simulink library "THB_fixed_T"  (Simulink 8.2)
settings: Solver=ode45  StartTime=0.0  StopTime=10.0  RelTol=1e-3
libraries: carnot x1
settings Model: Creator=lena.frank  LastModifiedBy=awohlfei

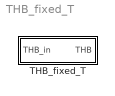
== system THB_fixed_T ==
  THB_fixed_T : Subsystem  InitFcn=load('THB.mat');  mask(set temperature in THB){t=60}
      mask prompts: t "temperature in degree Celsuis"
      mask help: Set a constant temperature in the thermo-hydraulic bus.
      mask Help: web(['file:///' fullfile(path_carnot('help'),'THB_fixed_T.html')],'-helpbrowser')

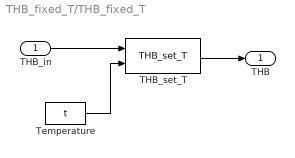
== system THB_fixed_T/THB_fixed_T ==
  THB_in : Inport
  THB_set_T : carnot/Source/Simple/THB_set_T
  Temperature : Constant  Value=t
  THB : Outport
  wires:
  Temperature/1 -> THB_set_T/2
  THB_in/1 -> THB_set_T/1
  THB_set_T/1 -> THB/1
